simulink model "robocup"  (Simulink 8.4)
settings: Solver=ode45  StartTime=0.0  StopTime=10.0  RelTol=1e-3
libraries: simulink x2

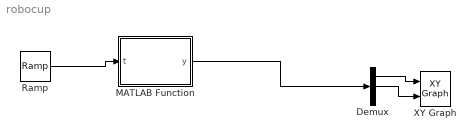
== system robocup ==
  Demux : Demux  Outputs=3
  MATLAB Function : MATLAB Function  TreatAsAtomicUnit=on
  Ramp : simulink/Sources/Ramp  slope=1  start=0  X0=0
  XY Graph : simulink/Sinks/XY Graph  xmin=-1  xmax=10  ymin=-1  ymax=10  st=-1
  wires:
  Ramp/1 -> MATLAB Function/1(t)
  MATLAB Function/1(y) -> Demux/1
  Demux/1 -> XY Graph/1
  Demux/2 -> XY Graph/2

== matlab function MATLAB Function ==
function y = fcn(t)
y = DiagonalPath(t)'
